simulink library "halin"  (R2021b)
settings: Solver=VariableStepAuto  StartTime=0.0  StopTime=10.0  RelTol=1e-3
undefined symbols (not defined in the file): KHAL_CAN1ABM1E2E_flg, KHAL_CAN1EPB1E2E_flg, KHAL_CAN1EPS1E2E_flg, KHAL_CAN1ESC1E2E_flg, KHAL_CAN1ESC5E2E_flg, KHAL_CAN3BMS1E2E_flg, KHAL_CAN3BMS6E2E_flg, KHAL_CAN3CCU1E2E_flg, KHAL_CAN3CCU2E2E_flg, KHAL_CAN3MCUNF1E2E_flg, KHAL_CAN3MCUNR1E2E_flg, KHAL_CAN3Shifter1E2E_flg, KHAL_CAN3Shifter2E2E_flg, KHAL_CAN6FCM2E2E_flg, KHAL_CAN6FCM4E2E_flg, TRUE
libraries: simulink x645, FVT_lib x207, hcu_lib x59
(part 13 of 23)

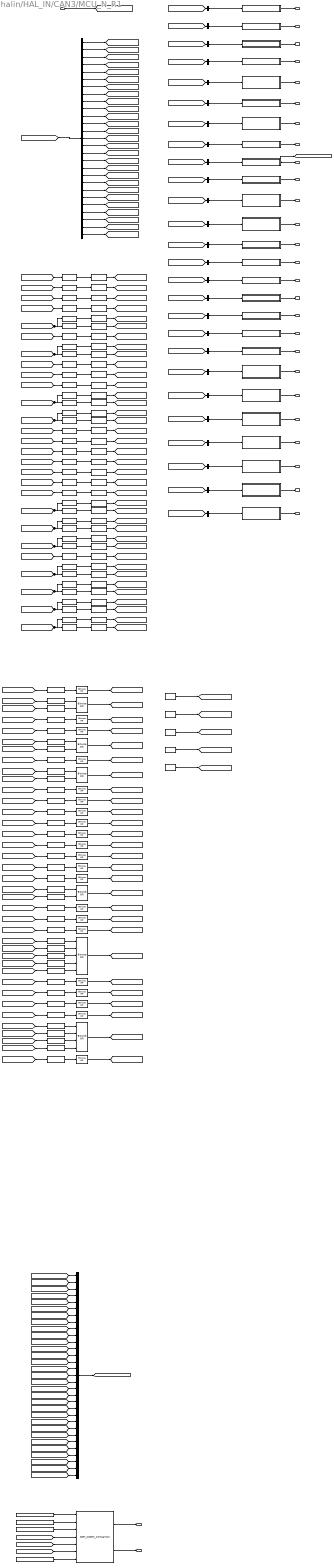
== system halin/HAL_IN/CAN3/MCU_N_R1 ==
  DT_CAN3_SG_MCU_N_R1 : Inport
  0x02 : Constant  Value=0x02
  0x78 : Constant  Value=0x78
  BitwiseAND{,1..37} (38 alike) : simulink/Logic and Bit Operations/Bitwise Operator  logicop=AND  UseBitMask=on  BitMask=0xFF  BitMaskRealWorld=Stored Integer
  BitwiseOR{,2..3,5,7..15,17..19,21..24,26} (21 alike) : simulink/Logic and Bit Operations/Bitwise Operator  logicop=OR  UseBitMask=off  BitMask=bin2dec('11011001')  BitMaskRealWorld=Stored Integer
  BitwiseOR{1,4,6,16} (4 alike) : simulink/Logic and Bit Operations/Bitwise Operator  logicop=OR  UseBitMask=off  NumInputPorts=2  BitMask=bin2dec('11011001')  BitMaskRealWorld=Stored Integer
  BitwiseOR20 : simulink/Logic and Bit Operations/Bitwise Operator  logicop=OR  UseBitMask=off  NumInputPorts=5  BitMask=bin2dec('11011001')  BitMaskRealWorld=Stored Integer
  BitwiseOR25 : simulink/Logic and Bit Operations/Bitwise Operator  logicop=OR  UseBitMask=off  NumInputPorts=4  BitMask=bin2dec('11011001')  BitMaskRealWorld=Stored Integer
  DDM_CS&RC_Comparison : FVT_lib/hal/DDM_CS&RC_Comparison  MsgCycleTime=10
  Data Type Conversion{,1..37} (38 alike) : DataTypeConversion  OutDataTypeStr=uint8
  KHAL_CAN3MCUNR1E2E_flg : Constant  Value=KHAL_CAN3MCUNR1E2E_flg
  LeftShift{,5,7,10..12,14} (7 alike) : ArithShift  BitShiftDirection=Left
  LeftShift1 : ArithShift  BitShiftNumber=1  BitShiftDirection=Left
  LeftShift13 : ArithShift  BitShiftNumber=7  BitShiftDirection=Left
  LeftShift15 : ArithShift  BitShiftNumber=1  BitShiftDirection=Left
  LeftShift2 : ArithShift  BitShiftNumber=2  BitShiftDirection=Left
  LeftShift3 : ArithShift  BitShiftNumber=5  BitShiftDirection=Left
  LeftShift4 : ArithShift  BitShiftNumber=6  BitShiftDirection=Left
  LeftShift6 : ArithShift  BitShiftNumber=4  BitShiftDirection=Left
  LeftShift8 : ArithShift  BitShiftNumber=3  BitShiftDirection=Left
  LeftShift9 : ArithShift  BitShiftNumber=4  BitShiftDirection=Left
  MCUWarnRNidec : Subsystem
  MessageRollingCounter : FVT_lib/hal/MessageRollingCounter  CounterMAX=14  task_time_ms=5  msg_time_ms=10
  Mux : Mux  Inputs=31
  RightShift{,2,4,6,10,14,16,18,20} (9 alike) : ArithShift  BitShiftNumber=8
  RightShift{1,3,5,7,11,15,17,19,21} (9 alike) : ArithShift
  RightShift12 : ArithShift  BitShiftNumber=4
  RightShift13 : ArithShift  BitShiftNumber=-4
  RightShift8 : ArithShift  BitShiftNumber=1
  RightShift9 : ArithShift  BitShiftNumber=-7
  RrActvDmpDisabStaNidec : Subsystem
  RrEDUDrtStaNidec : Subsystem
  RrEDUOpratingStaNidec : Subsystem
  RrEDURealTMTqNidec : Subsystem
  RrEDURotateDirctionNidec : Subsystem
  RrEDUTqReqFbkNidec : Subsystem
  RrMCU1ChksumNidec : Subsystem
  RrMCU1RolCntNidec : Subsystem
  RrMCUBATNidec : Subsystem
  RrMCUDCBusCurrNidec : Subsystem
  RrMCUDCBusVoltNidec : Subsystem
  RrMCUDischrgStaNidec : Subsystem
  RrMCUEnaStaNidec : Subsystem
  RrMCUErrNidec : Subsystem
  RrMCUIGNstaNidec : Subsystem
  RrMCUReady4PreNidec : Subsystem
  RrMCUReadyNidec : Subsystem
  RrMCUSysStaNidec : Subsystem
  RrMCUTempNidec : Subsystem
  RrMotorAvailTqNidec : Subsystem
  RrRegenAvailTqNidec : Subsystem
  RrTMSpdNidec : Subsystem
  RrTMTempNidec : Subsystem
  RrTMidNidec : Subsystem
  RrTMiqNidec : Subsystem
  bus_selector : BusSelector  OutputSignals=CAN3_MCUWarn_R_Nidec,CAN3_Rr_ActvDmpDisabSta_Nidec,CAN3_Rr_EDUDrtSta_Nidec,CAN3_Rr_EDUOpratingSta_Nidec,CAN3_Rr_EDURealTMTq_Nidec,CAN3_Rr_EDURotateDirction_Nidec,CAN3_Rr_EDUTqReqFbk_Nidec,CAN3_Rr_MCU1Chksum_Nidec,CAN3_Rr_MCU1RolCnt_Nidec,CAN3_Rr_MCUBAT_Nidec,CAN3_Rr_MCUDCBusCurr_Nidec,CAN3_Rr_MCUDCBusVolt_Nidec,CAN3_Rr_MCUDischrgSta_Nidec,CAN3_Rr_MCUEnaSta_Nidec,CAN3_Rr_MCUErr_Nidec,CAN3_Rr_MCUIGN_sta_Nidec,CAN3_Rr_MCUReady4Pre_Nidec,CAN3_Rr_MCUReady_Nidec,CAN3_Rr_MCUSysSta_Nidec,CAN3_Rr_MCUTemp_Nidec,CAN3_Rr_MotorAvailTq_Nidec,CAN3_Rr_RegenAvailTq_Nidec,CAN3_Rr_Reserved_bits_Nidec,CAN3_Rr_TMSpd_Nidec,CAN3_Rr_TMTemp_Nidec,CAN3_Rr_TMid_Nidec,CAN3_Rr_TMiq_Nidec
  bus_selector1 : BusSelector  OutputSignals=CAN3_MCUWarn_R_Nidec
  bus_selector10 : BusSelector  OutputSignals=CAN3_Rr_MCUBAT_Nidec
  bus_selector11 : BusSelector  OutputSignals=CAN3_Rr_MCUDCBusCurr_Nidec
  bus_selector12 : BusSelector  OutputSignals=CAN3_Rr_MCUDCBusVolt_Nidec
  bus_selector13 : BusSelector  OutputSignals=CAN3_Rr_MCUDischrgSta_Nidec
  bus_selector14 : BusSelector  OutputSignals=CAN3_Rr_MCUEnaSta_Nidec
  bus_selector15 : BusSelector  OutputSignals=CAN3_Rr_MCUErr_Nidec
  bus_selector16 : BusSelector  OutputSignals=CAN3_Rr_MCUIGN_sta_Nidec
  bus_selector17 : BusSelector  OutputSignals=CAN3_Rr_MCUReady4Pre_Nidec
  bus_selector18 : BusSelector  OutputSignals=CAN3_Rr_MCUReady_Nidec
  bus_selector19 : BusSelector  OutputSignals=CAN3_Rr_MCUSysSta_Nidec
  bus_selector2 : BusSelector  OutputSignals=CAN3_Rr_ActvDmpDisabSta_Nidec
  bus_selector20 : BusSelector  OutputSignals=CAN3_Rr_MCUTemp_Nidec
  bus_selector21 : BusSelector  OutputSignals=CAN3_Rr_MotorAvailTq_Nidec
  bus_selector22 : BusSelector  OutputSignals=CAN3_Rr_RegenAvailTq_Nidec
  bus_selector23 : BusSelector  OutputSignals=CAN3_Rr_TMSpd_Nidec
  bus_selector24 : BusSelector  OutputSignals=CAN3_Rr_TMTemp_Nidec
  bus_selector25 : BusSelector  OutputSignals=CAN3_Rr_TMid_Nidec
  bus_selector26 : BusSelector  OutputSignals=CAN3_Rr_TMiq_Nidec
  bus_selector3 : BusSelector  OutputSignals=CAN3_Rr_EDUDrtSta_Nidec
  bus_selector4 : BusSelector  OutputSignals=CAN3_Rr_EDUOpratingSta_Nidec
  bus_selector5 : BusSelector  OutputSignals=CAN3_Rr_EDURealTMTq_Nidec
  bus_selector6 : BusSelector  OutputSignals=CAN3_Rr_EDURotateDirction_Nidec
  bus_selector7 : BusSelector  OutputSignals=CAN3_Rr_EDUTqReqFbk_Nidec
  bus_selector8 : BusSelector  OutputSignals=CAN3_Rr_MCU1Chksum_Nidec
  bus_selector9 : BusSelector  OutputSignals=CAN3_Rr_MCU1RolCnt_Nidec
  constant{,1..4} (5 alike) : Constant  Value=0x0  OutDataTypeStr=uint8
  VHAL_MCUNR1CSErr_flg : Outport
  VHAL_MCUNR1RCErr_flg : Outport  Port=2
  VHAL_MCUWarnRNidec_enum : Outport  Port=3
  VHAL_RrActvDmpDisabStaNidec_flg : Outport  Port=4
  VHAL_RrEDUDrtStaNidec_flg : Outport  Port=5
  VHAL_RrEDUOpratingStaNidec_flg : Outport  Port=6
  VHAL_RrEDURealTMTqNidec_Nm : Outport  Port=7
  VHAL_RrEDURotateDirctionNidec_enum : Outport  Port=8
  VHAL_RrEDUTqReqFbkNidec_Nm : Outport  Port=9
  VHAL_RrMCU1ChksumNidec_enum : Outport  Port=10
  VHAL_RrMCU1RolCntNidec_enum : Outport  Port=11
  VHAL_RrMCUBATNidec_V : Outport  Port=12
  VHAL_RrMCUDCBusCurrNidec_A : Outport  Port=13
  VHAL_RrMCUDCBusVoltNidec_V : Outport  Port=14
  VHAL_RrMCUDischrgStaNidec_flg : Outport  Port=15
  VHAL_RrMCUEnaStaNidec_flg : Outport  Port=16
  VHAL_RrMCUErrNidec_enum : Outport  Port=17
  VHAL_RrMCUIGNstaNidec_flg : Outport  Port=18
  VHAL_RrMCUReady4PreNidec_flg : Outport  Port=19
  VHAL_RrMCUReadyNidec_flg : Outport  Port=20
  VHAL_RrMCUSysStaNidec_enum : Outport  Port=21
  VHAL_RrMCUTempNidec_C : Outport  Port=22
  VHAL_RrMotorAvailTqNidec_Nm : Outport  Port=23
  VHAL_RrRegenAvailTqNidec_Nm : Outport  Port=24
  VHAL_RrTMSpdNidec_rpm : Outport  Port=25
  VHAL_RrTMTempNidec_C : Outport  Port=26
  VHAL_RrTMidNidec_A : Outport  Port=27
  VHAL_RrTMiqNidec_A : Outport  Port=28
  wires:
  DT_CAN3_SG_MCU_N_R1/1 -> [DT_CAN3_SG_MCU_N_R1]
  [DT_CAN3_SG_MCU_N_R1] -> bus_selector/1
  bus_selector/1 -> [CAN3_MCUWarn_R_Nidec]  "<CAN3_MCUWarn_R_Nidec>"
  [CAN3_MCUWarn_R_Nidec] -> LeftShift/1
  LeftShift/1 -> BitwiseAND/1
  BitwiseAND/1 -> [Byte_1_CAN3_MCUWarn_R_Nidec]
  bus_selector/2 -> [CAN3_Rr_ActvDmpDisabSta_Nidec]  "<CAN3_Rr_ActvDmpDisabSta_Nidec>"
  [CAN3_Rr_ActvDmpDisabSta_Nidec] -> LeftShift1/1
  LeftShift1/1 -> BitwiseAND1/1
  BitwiseAND1/1 -> [Byte_25_CAN3_Rr_ActvDmpDisabSta_Nidec]
  bus_selector/3 -> [CAN3_Rr_EDUDrtSta_Nidec]  "<CAN3_Rr_EDUDrtSta_Nidec>"
  [CAN3_Rr_EDUDrtSta_Nidec] -> LeftShift2/1
  LeftShift2/1 -> BitwiseAND2/1
  BitwiseAND2/1 -> [Byte_25_CAN3_Rr_EDUDrtSta_Nidec]
  bus_selector/4 -> [CAN3_Rr_EDUOpratingSta_Nidec]  "<CAN3_Rr_EDUOpratingSta_Nidec>"
  [CAN3_Rr_EDUOpratingSta_Nidec] -> LeftShift3/1
  LeftShift3/1 -> BitwiseAND3/1
  BitwiseAND3/1 -> [Byte_30_CAN3_Rr_EDUOpratingSta_Nidec]
  bus_selector/5 -> [CAN3_Rr_EDURealTMTq_Nidec]  "<CAN3_Rr_EDURealTMTq_Nidec>"
  [CAN3_Rr_EDURealTMTq_Nidec] -> RightShift/1, RightShift1/1
  RightShift/1 -> BitwiseAND4/1
  BitwiseAND4/1 -> [Byte_28_CAN3_Rr_EDURealTMTq_Nidec]
  RightShift1/1 -> BitwiseAND5/1
  BitwiseAND5/1 -> [Byte_29_CAN3_Rr_EDURealTMTq_Nidec]
  bus_selector/6 -> [CAN3_Rr_EDURotateDirction_Nidec]  "<CAN3_Rr_EDURotateDirction_Nidec>"
  [CAN3_Rr_EDURotateDirction_Nidec] -> LeftShift4/1
  LeftShift4/1 -> BitwiseAND6/1
  BitwiseAND6/1 -> [Byte_30_CAN3_Rr_EDURotateDirction_Nidec]
  bus_selector/7 -> [CAN3_Rr_EDUTqReqFbk_Nidec]  "<CAN3_Rr_EDUTqReqFbk_Nidec>"
  [CAN3_Rr_EDUTqReqFbk_Nidec] -> RightShift2/1, RightShift3/1
  RightShift2/1 -> BitwiseAND7/1
  BitwiseAND7/1 -> [Byte_30_CAN3_Rr_EDUTqReqFbk_Nidec]
  RightShift3/1 -> BitwiseAND8/1
  BitwiseAND8/1 -> [Byte_31_CAN3_Rr_EDUTqReqFbk_Nidec]
  bus_selector/8 -> [CAN3_Rr_MCU1Chksum_Nidec]  "<CAN3_Rr_MCU1Chksum_Nidec>"
  [CAN3_Rr_MCU1Chksum_Nidec] -> LeftShift5/1
  LeftShift5/1 -> BitwiseAND9/1
  BitwiseAND9/1 -> [Byte_0_CAN3_Rr_MCU1Chksum_Nidec]
  bus_selector/9 -> [CAN3_Rr_MCU1RolCnt_Nidec]  "<CAN3_Rr_MCU1RolCnt_Nidec>"
  [CAN3_Rr_MCU1RolCnt_Nidec] -> LeftShift6/1
  LeftShift6/1 -> BitwiseAND10/1
  BitwiseAND10/1 -> [Byte_1_CAN3_Rr_MCU1RolCnt_Nidec]
  bus_selector/10 -> [CAN3_Rr_MCUBAT_Nidec]  "<CAN3_Rr_MCUBAT_Nidec>"
  [CAN3_Rr_MCUBAT_Nidec] -> LeftShift7/1
  LeftShift7/1 -> BitwiseAND11/1
  BitwiseAND11/1 -> [Byte_8_CAN3_Rr_MCUBAT_Nidec]
  bus_selector/11 -> [CAN3_Rr_MCUDCBusCurr_Nidec]  "<CAN3_Rr_MCUDCBusCurr_Nidec>"
  [CAN3_Rr_MCUDCBusCurr_Nidec] -> RightShift4/1, RightShift5/1
  RightShift4/1 -> BitwiseAND12/1
  BitwiseAND12/1 -> [Byte_21_CAN3_Rr_MCUDCBusCurr_Nidec]
  RightShift5/1 -> BitwiseAND13/1
  BitwiseAND13/1 -> [Byte_22_CAN3_Rr_MCUDCBusCurr_Nidec]
  bus_selector/12 -> [CAN3_Rr_MCUDCBusVolt_Nidec]  "<CAN3_Rr_MCUDCBusVolt_Nidec>"
  [CAN3_Rr_MCUDCBusVolt_Nidec] -> RightShift6/1, RightShift7/1
  RightShift6/1 -> BitwiseAND14/1
  BitwiseAND14/1 -> [Byte_23_CAN3_Rr_MCUDCBusVolt_Nidec]
  RightShift7/1 -> BitwiseAND15/1
  BitwiseAND15/1 -> [Byte_24_CAN3_Rr_MCUDCBusVolt_Nidec]
  bus_selector/13 -> [CAN3_Rr_MCUDischrgSta_Nidec]  "<CAN3_Rr_MCUDischrgSta_Nidec>"
  [CAN3_Rr_MCUDischrgSta_Nidec] -> LeftShift8/1
  LeftShift8/1 -> BitwiseAND16/1
  BitwiseAND16/1 -> [Byte_25_CAN3_Rr_MCUDischrgSta_Nidec]
  bus_selector/14 -> [CAN3_Rr_MCUEnaSta_Nidec]  "<CAN3_Rr_MCUEnaSta_Nidec>"
  [CAN3_Rr_MCUEnaSta_Nidec] -> LeftShift9/1
  LeftShift9/1 -> BitwiseAND17/1
  BitwiseAND17/1 -> [Byte_30_CAN3_Rr_MCUEnaSta_Nidec]
  bus_selector/15 -> [CAN3_Rr_MCUErr_Nidec]  "<CAN3_Rr_MCUErr_Nidec>"
  [CAN3_Rr_MCUErr_Nidec] -> LeftShift10/1
  LeftShift10/1 -> BitwiseAND18/1
  BitwiseAND18/1 -> [Byte_17_CAN3_Rr_MCUErr_Nidec]
  bus_selector/16 -> [CAN3_Rr_MCUIGN_sta_Nidec]  "<CAN3_Rr_MCUIGN_sta_Nidec>"
  [CAN3_Rr_MCUIGN_sta_Nidec] -> LeftShift11/1
  LeftShift11/1 -> BitwiseAND19/1
  BitwiseAND19/1 -> [Byte_9_CAN3_Rr_MCUIGN_sta_Nidec]
  bus_selector/17 -> [CAN3_Rr_MCUReady4Pre_Nidec]  "<CAN3_Rr_MCUReady4Pre_Nidec>"
  [CAN3_Rr_MCUReady4Pre_Nidec] -> LeftShift12/1
  LeftShift12/1 -> BitwiseAND20/1
  BitwiseAND20/1 -> [Byte_25_CAN3_Rr_MCUReady4Pre_Nidec]
  bus_selector/18 -> [CAN3_Rr_MCUReady_Nidec]  "<CAN3_Rr_MCUReady_Nidec>"
  [CAN3_Rr_MCUReady_Nidec] -> LeftShift13/1
  LeftShift13/1 -> BitwiseAND21/1
  BitwiseAND21/1 -> [Byte_25_CAN3_Rr_MCUReady_Nidec]
  bus_selector/19 -> [CAN3_Rr_MCUSysSta_Nidec]  "<CAN3_Rr_MCUSysSta_Nidec>"
  [CAN3_Rr_MCUSysSta_Nidec] -> LeftShift14/1
  LeftShift14/1 -> BitwiseAND22/1
  BitwiseAND22/1 -> [Byte_7_CAN3_Rr_MCUSysSta_Nidec]
  bus_selector/20 -> [CAN3_Rr_MCUTemp_Nidec]  "<CAN3_Rr_MCUTemp_Nidec>"
  [CAN3_Rr_MCUTemp_Nidec] -> RightShift8/1, RightShift9/1
  RightShift8/1 -> BitwiseAND23/1
  BitwiseAND23/1 -> [Byte_20_CAN3_Rr_MCUTemp_Nidec]
  RightShift9/1 -> BitwiseAND24/1
  BitwiseAND24/1 -> [Byte_21_CAN3_Rr_MCUTemp_Nidec]
  bus_selector/21 -> [CAN3_Rr_MotorAvailTq_Nidec]  "<CAN3_Rr_MotorAvailTq_Nidec>"
  [CAN3_Rr_MotorAvailTq_Nidec] -> RightShift10/1, RightShift11/1
  RightShift10/1 -> BitwiseAND25/1
  BitwiseAND25/1 -> [Byte_11_CAN3_Rr_MotorAvailTq_Nidec]
  RightShift11/1 -> BitwiseAND26/1
  BitwiseAND26/1 -> [Byte_12_CAN3_Rr_MotorAvailTq_Nidec]
  bus_selector/22 -> [CAN3_Rr_RegenAvailTq_Nidec]  "<CAN3_Rr_RegenAvailTq_Nidec>"
  [CAN3_Rr_RegenAvailTq_Nidec] -> RightShift12/1, RightShift13/1
  RightShift12/1 -> BitwiseAND27/1
  BitwiseAND27/1 -> [Byte_10_CAN3_Rr_RegenAvailTq_Nidec]
  RightShift13/1 -> BitwiseAND28/1
  BitwiseAND28/1 -> [Byte_11_CAN3_Rr_RegenAvailTq_Nidec]
  bus_selector/23 -> [CAN3_Rr_Reserved_bits_Nidec]  "<CAN3_Rr_Reserved_bits_Nidec>"
  [CAN3_Rr_Reserved_bits_Nidec] -> LeftShift15/1
  LeftShift15/1 -> BitwiseAND29/1
  BitwiseAND29/1 -> [Byte_9_CAN3_Rr_Reserved_bits_Nidec]
  bus_selector/24 -> [CAN3_Rr_TMSpd_Nidec]  "<CAN3_Rr_TMSpd_Nidec>"
  [CAN3_Rr_TMSpd_Nidec] -> RightShift14/1, RightShift15/1
  RightShift14/1 -> BitwiseAND30/1
  BitwiseAND30/1 -> [Byte_26_CAN3_Rr_TMSpd_Nidec]
  RightShift15/1 -> BitwiseAND31/1
  BitwiseAND31/1 -> [Byte_27_CAN3_Rr_TMSpd_Nidec]
  bus_selector/25 -> [CAN3_Rr_TMTemp_Nidec]  "<CAN3_Rr_TMTemp_Nidec>"
  [CAN3_Rr_TMTemp_Nidec] -> RightShift16/1, RightShift17/1
  RightShift16/1 -> BitwiseAND32/1
  BitwiseAND32/1 -> [Byte_18_CAN3_Rr_TMTemp_Nidec]
  RightShift17/1 -> BitwiseAND33/1
  BitwiseAND33/1 -> [Byte_19_CAN3_Rr_TMTemp_Nidec]
  bus_selector/26 -> [CAN3_Rr_TMid_Nidec]  "<CAN3_Rr_TMid_Nidec>"
  [CAN3_Rr_TMid_Nidec] -> RightShift18/1, RightShift19/1
  RightShift18/1 -> BitwiseAND34/1
  BitwiseAND34/1 -> [Byte_15_CAN3_Rr_TMid_Nidec]
  RightShift19/1 -> BitwiseAND35/1
  BitwiseAND35/1 -> [Byte_16_CAN3_Rr_TMid_Nidec]
  bus_selector/27 -> [CAN3_Rr_TMiq_Nidec]  "<CAN3_Rr_TMiq_Nidec>"
  [CAN3_Rr_TMiq_Nidec] -> RightShift20/1, RightShift21/1
  RightShift20/1 -> BitwiseAND36/1
  BitwiseAND36/1 -> [Byte_13_CAN3_Rr_TMiq_Nidec]
  RightShift21/1 -> BitwiseAND37/1
  BitwiseAND37/1 -> [Byte_14_CAN3_Rr_TMiq_Nidec]
  Data Type Conversion/1 -> BitwiseOR/1
  [Byte_0_CAN3_Rr_MCU1Chksum_Nidec] -> Data Type Conversion/1
  BitwiseOR/1 -> [Byte_0]
  Data Type Conversion1/1 -> BitwiseOR1/1
  [Byte_1_CAN3_MCUWarn_R_Nidec] -> Data Type Conversion1/1
  Data Type Conversion2/1 -> BitwiseOR1/2
  [Byte_1_CAN3_Rr_MCU1RolCnt_Nidec] -> Data Type Conversion2/1
  BitwiseOR1/1 -> [Byte_1]
  constant/1 -> [Byte_2]
  constant1/1 -> [Byte_3]
  constant2/1 -> [Byte_4]
  constant3/1 -> [Byte_5]
  constant4/1 -> [Byte_6]
  Data Type Conversion3/1 -> BitwiseOR2/1
  [Byte_7_CAN3_Rr_MCUSysSta_Nidec] -> Data Type Conversion3/1
  BitwiseOR2/1 -> [Byte_7]
  Data Type Conversion4/1 -> BitwiseOR3/1
  [Byte_8_CAN3_Rr_MCUBAT_Nidec] -> Data Type Conversion4/1
  BitwiseOR3/1 -> [Byte_8]
  Data Type Conversion5/1 -> BitwiseOR4/1
  [Byte_9_CAN3_Rr_MCUIGN_sta_Nidec] -> Data Type Conversion5/1
  Data Type Conversion6/1 -> BitwiseOR4/2
  [Byte_9_CAN3_Rr_Reserved_bits_Nidec] -> Data Type Conversion6/1
  BitwiseOR4/1 -> [Byte_9]
  Data Type Conversion7/1 -> BitwiseOR5/1
  [Byte_10_CAN3_Rr_RegenAvailTq_Nidec] -> Data Type Conversion7/1
  BitwiseOR5/1 -> [Byte_10]
  Data Type Conversion8/1 -> BitwiseOR6/1
  [Byte_11_CAN3_Rr_MotorAvailTq_Nidec] -> Data Type Conversion8/1
  Data Type Conversion9/1 -> BitwiseOR6/2
  [Byte_11_CAN3_Rr_RegenAvailTq_Nidec] -> Data Type Conversion9/1
  BitwiseOR6/1 -> [Byte_11]
  Data Type Conversion10/1 -> BitwiseOR7/1
  [Byte_12_CAN3_Rr_MotorAvailTq_Nidec] -> Data Type Conversion10/1
  BitwiseOR7/1 -> [Byte_12]
  Data Type Conversion11/1 -> BitwiseOR8/1
  [Byte_13_CAN3_Rr_TMiq_Nidec] -> Data Type Conversion11/1
  BitwiseOR8/1 -> [Byte_13]
  Data Type Conversion12/1 -> BitwiseOR9/1
  [Byte_14_CAN3_Rr_TMiq_Nidec] -> Data Type Conversion12/1
  BitwiseOR9/1 -> [Byte_14]
  Data Type Conversion13/1 -> BitwiseOR10/1
  [Byte_15_CAN3_Rr_TMid_Nidec] -> Data Type Conversion13/1
  BitwiseOR10/1 -> [Byte_15]
  Data Type Conversion14/1 -> BitwiseOR11/1
  [Byte_16_CAN3_Rr_TMid_Nidec] -> Data Type Conversion14/1
  BitwiseOR11/1 -> [Byte_16]
  Data Type Conversion15/1 -> BitwiseOR12/1
  [Byte_17_CAN3_Rr_MCUErr_Nidec] -> Data Type Conversion15/1
  BitwiseOR12/1 -> [Byte_17]
  Data Type Conversion16/1 -> BitwiseOR13/1
  [Byte_18_CAN3_Rr_TMTemp_Nidec] -> Data Type Conversion16/1
  BitwiseOR13/1 -> [Byte_18]
  Data Type Conversion17/1 -> BitwiseOR14/1
  [Byte_19_CAN3_Rr_TMTemp_Nidec] -> Data Type Conversion17/1
  BitwiseOR14/1 -> [Byte_19]
  Data Type Conversion18/1 -> BitwiseOR15/1
  [Byte_20_CAN3_Rr_MCUTemp_Nidec] -> Data Type Conversion18/1
  BitwiseOR15/1 -> [Byte_20]
  Data Type Conversion19/1 -> BitwiseOR16/1
  [Byte_21_CAN3_Rr_MCUDCBusCurr_Nidec] -> Data Type Conversion19/1
  Data Type Conversion20/1 -> BitwiseOR16/2
  [Byte_21_CAN3_Rr_MCUTemp_Nidec] -> Data Type Conversion20/1
  BitwiseOR16/1 -> [Byte_21]
  Data Type Conversion21/1 -> BitwiseOR17/1
  [Byte_22_CAN3_Rr_MCUDCBusCurr_Nidec] -> Data Type Conversion21/1
  BitwiseOR17/1 -> [Byte_22]
  Data Type Conversion22/1 -> BitwiseOR18/1
  [Byte_23_CAN3_Rr_MCUDCBusVolt_Nidec] -> Data Type Conversion22/1
  BitwiseOR18/1 -> [Byte_23]
  Data Type Conversion23/1 -> BitwiseOR19/1
  [Byte_24_CAN3_Rr_MCUDCBusVolt_Nidec] -> Data Type Conversion23/1
  BitwiseOR19/1 -> [Byte_24]
  Data Type Conversion24/1 -> BitwiseOR20/1
  [Byte_25_CAN3_Rr_ActvDmpDisabSta_Nidec] -> Data Type Conversion24/1
  Data Type Conversion25/1 -> BitwiseOR20/2
  [Byte_25_CAN3_Rr_EDUDrtSta_Nidec] -> Data Type Conversion25/1
  Data Type Conversion26/1 -> BitwiseOR20/3
  [Byte_25_CAN3_Rr_MCUDischrgSta_Nidec] -> Data Type Conversion26/1
  Data Type Conversion27/1 -> BitwiseOR20/4
  [Byte_25_CAN3_Rr_MCUReady4Pre_Nidec] -> Data Type Conversion27/1
  Data Type Conversion28/1 -> BitwiseOR20/5
  [Byte_25_CAN3_Rr_MCUReady_Nidec] -> Data Type Conversion28/1
  BitwiseOR20/1 -> [Byte_25]
  Data Type Conversion29/1 -> BitwiseOR21/1
  [Byte_26_CAN3_Rr_TMSpd_Nidec] -> Data Type Conversion29/1
  BitwiseOR21/1 -> [Byte_26]
  Data Type Conversion30/1 -> BitwiseOR22/1
  [Byte_27_CAN3_Rr_TMSpd_Nidec] -> Data Type Conversion30/1
  BitwiseOR22/1 -> [Byte_27]
  Data Type Conversion31/1 -> BitwiseOR23/1
  [Byte_28_CAN3_Rr_EDURealTMTq_Nidec] -> Data Type Conversion31/1
  BitwiseOR23/1 -> [Byte_28]
  Data Type Conversion32/1 -> BitwiseOR24/1
  [Byte_29_CAN3_Rr_EDURealTMTq_Nidec] -> Data Type Conversion32/1
  BitwiseOR24/1 -> [Byte_29]
  Data Type Conversion33/1 -> BitwiseOR25/1
  [Byte_30_CAN3_Rr_EDUOpratingSta_Nidec] -> Data Type Conversion33/1
  Data Type Conversion34/1 -> BitwiseOR25/2
  [Byte_30_CAN3_Rr_EDURotateDirction_Nidec] -> Data Type Conversion34/1
  Data Type Conversion35/1 -> BitwiseOR25/3
  [Byte_30_CAN3_Rr_EDUTqReqFbk_Nidec] -> Data Type Conversion35/1
  Data Type Conversion36/1 -> BitwiseOR25/4
  [Byte_30_CAN3_Rr_MCUEnaSta_Nidec] -> Data Type Conversion36/1
  BitwiseOR25/1 -> [Byte_30]
  Data Type Conversion37/1 -> BitwiseOR26/1
  [Byte_31_CAN3_Rr_EDUTqReqFbk_Nidec] -> Data Type Conversion37/1
  BitwiseOR26/1 -> [Byte_31]
  [Byte_1] -> Mux/1
  [Byte_2] -> Mux/2
  [Byte_3] -> Mux/3
  [Byte_4] -> Mux/4
  [Byte_5] -> Mux/5
  [Byte_6] -> Mux/6
  [Byte_7] -> Mux/7
  [Byte_8] -> Mux/8
  [Byte_9] -> Mux/9
  [Byte_10] -> Mux/10
  [Byte_11] -> Mux/11
  [Byte_12] -> Mux/12
  [Byte_13] -> Mux/13
  [Byte_14] -> Mux/14
  [Byte_15] -> Mux/15
  [Byte_16] -> Mux/16
  [Byte_17] -> Mux/17
  [Byte_18] -> Mux/18
  [Byte_19] -> Mux/19
  [Byte_20] -> Mux/20
  [Byte_21] -> Mux/21
  [Byte_22] -> Mux/22
  [Byte_23] -> Mux/23
  [Byte_24] -> Mux/24
  [Byte_25] -> Mux/25
  [Byte_26] -> Mux/26
  [Byte_27] -> Mux/27
  [Byte_28] -> Mux/28
  [Byte_29] -> Mux/29
  [Byte_30] -> Mux/30
  [Byte_31] -> Mux/31
  Mux/1 -> [VHAL_CAN3MCUNR1noCS_raw]
  KHAL_CAN3MCUNR1E2E_flg/1 -> DDM_CS&RC_Comparison/1
  0x78/1 -> DDM_CS&RC_Comparison/2
  0x02/1 -> DDM_CS&RC_Comparison/3
  [VHAL_CAN3MCUNR1noCS_raw] -> DDM_CS&RC_Comparison/4
  [Byte_0] -> DDM_CS&RC_Comparison/5
  [RC_ECU] -> DDM_CS&RC_Comparison/6
  MessageRollingCounter/1 -> DDM_CS&RC_Comparison/7
  DDM_CS&RC_Comparison/1 -> VHAL_MCUNR1CSErr_flg/1
  DDM_CS&RC_Comparison/2 -> VHAL_MCUNR1RCErr_flg/1
  [DT_CAN3_SG_MCU_N_R1] -> bus_selector1/1
  bus_selector1/1 -> MCUWarnRNidec/1(MCUWarn_R_Nidec)  "<CAN3_MCUWarn_R_Nidec>"
  MCUWarnRNidec/1(VHAL_MCUWarnRNidec_enum) -> VHAL_MCUWarnRNidec_enum/1
  [DT_CAN3_SG_MCU_N_R1] -> bus_selector2/1
  bus_selector2/1 -> RrActvDmpDisabStaNidec/1(Rr_ActvDmpDisabSta_Nidec)  "<CAN3_Rr_ActvDmpDisabSta_Nidec>"
  RrActvDmpDisabStaNidec/1(VHAL_RrActvDmpDisabStaNidec_flg) -> VHAL_RrActvDmpDisabStaNidec_flg/1
  [DT_CAN3_SG_MCU_N_R1] -> bus_selector3/1
  bus_selector3/1 -> RrEDUDrtStaNidec/1(Rr_EDUDrtSta_Nidec)  "<CAN3_Rr_EDUDrtSta_Nidec>"
  RrEDUDrtStaNidec/1(VHAL_RrEDUDrtStaNidec_flg) -> VHAL_RrEDUDrtStaNidec_flg/1
  [DT_CAN3_SG_MCU_N_R1] -> bus_selector4/1
  bus_selector4/1 -> RrEDUOpratingStaNidec/1(Rr_EDUOpratingSta_Nidec)  "<CAN3_Rr_EDUOpratingSta_Nidec>"
  RrEDUOpratingStaNidec/1(VHAL_RrEDUOpratingStaNidec_flg) -> VHAL_RrEDUOpratingStaNidec_flg/1
  [DT_CAN3_SG_MCU_N_R1] -> bus_selector5/1
  bus_selector5/1 -> RrEDURealTMTqNidec/1(Rr_EDURealTMTq_Nidec)  "<CAN3_Rr_EDURealTMTq_Nidec>"
  RrEDURealTMTqNidec/1(VHAL_RrEDURealTMTqNidec_Nm) -> VHAL_RrEDURealTMTqNidec_Nm/1
  [DT_CAN3_SG_MCU_N_R1] -> bus_selector6/1
  bus_selector6/1 -> RrEDURotateDirctionNidec/1(Rr_EDURotateDirction_Nidec)  "<CAN3_Rr_EDURotateDirction_Nidec>"
  RrEDURotateDirctionNidec/1(VHAL_RrEDURotateDirctionNidec_enum) -> VHAL_RrEDURotateDirctionNidec_enum/1
  [DT_CAN3_SG_MCU_N_R1] -> bus_selector7/1
  bus_selector7/1 -> RrEDUTqReqFbkNidec/1(Rr_EDUTqReqFbk_Nidec)  "<CAN3_Rr_EDUTqReqFbk_Nidec>"
  RrEDUTqReqFbkNidec/1(VHAL_RrEDUTqReqFbkNidec_Nm) -> VHAL_RrEDUTqReqFbkNidec_Nm/1
  [DT_CAN3_SG_MCU_N_R1] -> bus_selector8/1
  bus_selector8/1 -> RrMCU1ChksumNidec/1(Rr_MCU1Chksum_Nidec)  "<CAN3_Rr_MCU1Chksum_Nidec>"
  RrMCU1ChksumNidec/1(VHAL_RrMCU1ChksumNidec_enum) -> VHAL_RrMCU1ChksumNidec_enum/1
  [DT_CAN3_SG_MCU_N_R1] -> bus_selector9/1
  bus_selector9/1 -> RrMCU1RolCntNidec/1(Rr_MCU1RolCnt_Nidec)  "<CAN3_Rr_MCU1RolCnt_Nidec>"
  RrMCU1RolCntNidec/1(VHAL_RrMCU1RolCntNidec_enum) -> VHAL_RrMCU1RolCntNidec_enum/1, [RC_ECU]
  [DT_CAN3_SG_MCU_N_R1] -> bus_selector10/1
  bus_selector10/1 -> RrMCUBATNidec/1(Rr_MCUBAT_Nidec)  "<CAN3_Rr_MCUBAT_Nidec>"
  RrMCUBATNidec/1(VHAL_RrMCUBATNidec_V) -> VHAL_RrMCUBATNidec_V/1
  [DT_CAN3_SG_MCU_N_R1] -> bus_selector11/1
  bus_selector11/1 -> RrMCUDCBusCurrNidec/1(Rr_MCUDCBusCurr_Nidec)  "<CAN3_Rr_MCUDCBusCurr_Nidec>"
  RrMCUDCBusCurrNidec/1(VHAL_RrMCUDCBusCurrNidec_A) -> VHAL_RrMCUDCBusCurrNidec_A/1
  [DT_CAN3_SG_MCU_N_R1] -> bus_selector12/1
  bus_selector12/1 -> RrMCUDCBusVoltNidec/1(Rr_MCUDCBusVolt_Nidec)  "<CAN3_Rr_MCUDCBusVolt_Nidec>"
  RrMCUDCBusVoltNidec/1(VHAL_RrMCUDCBusVoltNidec_V) -> VHAL_RrMCUDCBusVoltNidec_V/1
  [DT_CAN3_SG_MCU_N_R1] -> bus_selector13/1
  bus_selector13/1 -> RrMCUDischrgStaNidec/1(Rr_MCUDischrgSta_Nidec)  "<CAN3_Rr_MCUDischrgSta_Nidec>"
  RrMCUDischrgStaNidec/1(VHAL_RrMCUDischrgStaNidec_flg) -> VHAL_RrMCUDischrgStaNidec_flg/1
  [DT_CAN3_SG_MCU_N_R1] -> bus_selector14/1
  bus_selector14/1 -> RrMCUEnaStaNidec/1(Rr_MCUEnaSta_Nidec)  "<CAN3_Rr_MCUEnaSta_Nidec>"
  RrMCUEnaStaNidec/1(VHAL_RrMCUEnaStaNidec_flg) -> VHAL_RrMCUEnaStaNidec_flg/1
  [DT_CAN3_SG_MCU_N_R1] -> bus_selector15/1
  bus_selector15/1 -> RrMCUErrNidec/1(Rr_MCUErr_Nidec)  "<CAN3_Rr_MCUErr_Nidec>"
  RrMCUErrNidec/1(VHAL_RrMCUErrNidec_enum) -> VHAL_RrMCUErrNidec_enum/1
  [DT_CAN3_SG_MCU_N_R1] -> bus_selector16/1
  bus_selector16/1 -> RrMCUIGNstaNidec/1(Rr_MCUIGN_sta_Nidec)  "<CAN3_Rr_MCUIGN_sta_Nidec>"
  RrMCUIGNstaNidec/1(VHAL_RrMCUIGNstaNidec_flg) -> VHAL_RrMCUIGNstaNidec_flg/1
  [DT_CAN3_SG_MCU_N_R1] -> bus_selector17/1
  bus_selector17/1 -> RrMCUReady4PreNidec/1(Rr_MCUReady4Pre_Nidec)  "<CAN3_Rr_MCUReady4Pre_Nidec>"
  RrMCUReady4PreNidec/1(VHAL_RrMCUReady4PreNidec_flg) -> VHAL_RrMCUReady4PreNidec_flg/1
  [DT_CAN3_SG_MCU_N_R1] -> bus_selector18/1
  bus_selector18/1 -> RrMCUReadyNidec/1(Rr_MCUReady_Nidec)  "<CAN3_Rr_MCUReady_Nidec>"
  RrMCUReadyNidec/1(VHAL_RrMCUReadyNidec_flg) -> VHAL_RrMCUReadyNidec_flg/1
  [DT_CAN3_SG_MCU_N_R1] -> bus_selector19/1
  bus_selector19/1 -> RrMCUSysStaNidec/1(Rr_MCUSysSta_Nidec)  "<CAN3_Rr_MCUSysSta_Nidec>"
  RrMCUSysStaNidec/1(VHAL_RrMCUSysStaNidec_enum) -> VHAL_RrMCUSysStaNidec_enum/1
  [DT_CAN3_SG_MCU_N_R1] -> bus_selector20/1
  bus_selector20/1 -> RrMCUTempNidec/1(Rr_MCUTemp_Nidec)  "<CAN3_Rr_MCUTemp_Nidec>"
  RrMCUTempNidec/1(VHAL_RrMCUTempNidec_C) -> VHAL_RrMCUTempNidec_C/1
  [DT_CAN3_SG_MCU_N_R1] -> bus_selector21/1
  bus_selector21/1 -> RrMotorAvailTqNidec/1(Rr_MotorAvailTq_Nidec)  "<CAN3_Rr_MotorAvailTq_Nidec>"
  RrMotorAvailTqNidec/1(VHAL_RrMotorAvailTqNidec_Nm) -> VHAL_RrMotorAvailTqNidec_Nm/1
  [DT_CAN3_SG_MCU_N_R1] -> bus_selector22/1
  bus_selector22/1 -> RrRegenAvailTqNidec/1(Rr_RegenAvailTq_Nidec)  "<CAN3_Rr_RegenAvailTq_Nidec>"
  RrRegenAvailTqNidec/1(VHAL_RrRegenAvailTqNidec_Nm) -> VHAL_RrRegenAvailTqNidec_Nm/1
  [DT_CAN3_SG_MCU_N_R1] -> bus_selector23/1
  bus_selector23/1 -> RrTMSpdNidec/1(Rr_TMSpd_Nidec)  "<CAN3_Rr_TMSpd_Nidec>"
  RrTMSpdNidec/1(VHAL_RrTMSpdNidec_rpm) -> VHAL_RrTMSpdNidec_rpm/1
  [DT_CAN3_SG_MCU_N_R1] -> bus_selector24/1
  bus_selector24/1 -> RrTMTempNidec/1(Rr_TMTemp_Nidec)  "<CAN3_Rr_TMTemp_Nidec>"
  RrTMTempNidec/1(VHAL_RrTMTempNidec_C) -> VHAL_RrTMTempNidec_C/1
  [DT_CAN3_SG_MCU_N_R1] -> bus_selector25/1
  bus_selector25/1 -> RrTMidNidec/1(Rr_TMid_Nidec)  "<CAN3_Rr_TMid_Nidec>"
  RrTMidNidec/1(VHAL_RrTMidNidec_A) -> VHAL_RrTMidNidec_A/1
  [DT_CAN3_SG_MCU_N_R1] -> bus_selector26/1
  bus_selector26/1 -> RrTMiqNidec/1(Rr_TMiq_Nidec)  "<CAN3_Rr_TMiq_Nidec>"
  RrTMiqNidec/1(VHAL_RrTMiqNidec_A) -> VHAL_RrTMiqNidec_A/1

== system halin/HAL_IN/CAN3/MCU_N_R2 ==
  DT_CAN3_SG_MCU_N_R2 : Inport
  RrCoolanttempReqNidec : Subsystem
  RrEOPSpdSetNidec : Subsystem
  RrFailcode1Nidec : Subsystem
  RrFailcode2Nidec : Subsystem
  RrFailcodehistory1Nidec : Subsystem
  RrFailcodehistory2Nidec : Subsystem
  RrLLCTempNidec : Subsystem
  RrLLCflowReqNidec : Subsystem
  RrMCUTempWarnNidec : Subsystem
  RrTMTempWarnNidec : Subsystem
  bus_selector : BusSelector  OutputSignals=CAN3_Rr_CoolanttempReq_Nidec
  bus_selector1 : BusSelector  OutputSignals=CAN3_Rr_EOP_SpdSet_Nidec
  bus_selector2 : BusSelector  OutputSignals=CAN3_Rr_Failcode1_Nidec
  bus_selector3 : BusSelector  OutputSignals=CAN3_Rr_Failcode2_Nidec
  bus_selector4 : BusSelector  OutputSignals=CAN3_Rr_Failcodehistory1_Nidec
  bus_selector5 : BusSelector  OutputSignals=CAN3_Rr_Failcodehistory2_Nidec
  bus_selector6 : BusSelector  OutputSignals=CAN3_Rr_LLCTemp_Nidec
  bus_selector7 : BusSelector  OutputSignals=CAN3_Rr_LLCflowReq_Nidec
  bus_selector8 : BusSelector  OutputSignals=CAN3_Rr_MCUTempWarn_Nidec
  bus_selector9 : BusSelector  OutputSignals=CAN3_Rr_TMTempWarn_Nidec
  VHAL_RrCoolanttempReqNidec_cnt : Outport
  VHAL_RrEOPSpdSetNidec_rpm : Outport  Port=2
  VHAL_RrFailcode1Nidec_enum : Outport  Port=3
  VHAL_RrFailcode2Nidec_enum : Outport  Port=4
  VHAL_RrFailcodehistory1Nidec_enum : Outport  Port=5
  VHAL_RrFailcodehistory2Nidec_enum : Outport  Port=6
  VHAL_RrLLCTempNidec_C : Outport  Port=7
  VHAL_RrLLCflowReqNidec_Lpmin : Outport  Port=8
  VHAL_RrMCUTempWarnNidec_enum : Outport  Port=9
  VHAL_RrTMTempWarnNidec_enum : Outport  Port=10
  wires:
  DT_CAN3_SG_MCU_N_R2/1 -> [DT_CAN3_SG_MCU_N_R2]
  [DT_CAN3_SG_MCU_N_R2] -> bus_selector/1
  bus_selector/1 -> RrCoolanttempReqNidec/1(Rr_CoolanttempReq_Nidec)  "<CAN3_Rr_CoolanttempReq_Nidec>"
  RrCoolanttempReqNidec/1(VHAL_RrCoolanttempReqNidec_cnt) -> VHAL_RrCoolanttempReqNidec_cnt/1
  [DT_CAN3_SG_MCU_N_R2] -> bus_selector1/1
  bus_selector1/1 -> RrEOPSpdSetNidec/1(Rr_EOP_SpdSet_Nidec)  "<CAN3_Rr_EOP_SpdSet_Nidec>"
  RrEOPSpdSetNidec/1(VHAL_RrEOPSpdSetNidec_rpm) -> VHAL_RrEOPSpdSetNidec_rpm/1
  [DT_CAN3_SG_MCU_N_R2] -> bus_selector2/1
  bus_selector2/1 -> RrFailcode1Nidec/1(Rr_Failcode1_Nidec)  "<CAN3_Rr_Failcode1_Nidec>"
  RrFailcode1Nidec/1(VHAL_RrFailcode1Nidec_enum) -> VHAL_RrFailcode1Nidec_enum/1
  [DT_CAN3_SG_MCU_N_R2] -> bus_selector3/1
  bus_selector3/1 -> RrFailcode2Nidec/1(Rr_Failcode2_Nidec)  "<CAN3_Rr_Failcode2_Nidec>"
  RrFailcode2Nidec/1(VHAL_RrFailcode2Nidec_enum) -> VHAL_RrFailcode2Nidec_enum/1
  [DT_CAN3_SG_MCU_N_R2] -> bus_selector4/1
  bus_selector4/1 -> RrFailcodehistory1Nidec/1(Rr_Failcodehistory1_Nidec)  "<CAN3_Rr_Failcodehistory1_Nidec>"
  RrFailcodehistory1Nidec/1(VHAL_RrFailcodehistory1Nidec_enum) -> VHAL_RrFailcodehistory1Nidec_enum/1
  [DT_CAN3_SG_MCU_N_R2] -> bus_selector5/1
  bus_selector5/1 -> RrFailcodehistory2Nidec/1(Rr_Failcodehistory2_Nidec)  "<CAN3_Rr_Failcodehistory2_Nidec>"
  RrFailcodehistory2Nidec/1(VHAL_RrFailcodehistory2Nidec_enum) -> VHAL_RrFailcodehistory2Nidec_enum/1
  [DT_CAN3_SG_MCU_N_R2] -> bus_selector6/1
  bus_selector6/1 -> RrLLCTempNidec/1(Rr_LLCTemp_Nidec)  "<CAN3_Rr_LLCTemp_Nidec>"
  RrLLCTempNidec/1(VHAL_RrLLCTempNidec_C) -> VHAL_RrLLCTempNidec_C/1
  [DT_CAN3_SG_MCU_N_R2] -> bus_selector7/1
  bus_selector7/1 -> RrLLCflowReqNidec/1(Rr_LLCflowReq_Nidec)  "<CAN3_Rr_LLCflowReq_Nidec>"
  RrLLCflowReqNidec/1(VHAL_RrLLCflowReqNidec_Lpmin) -> VHAL_RrLLCflowReqNidec_Lpmin/1
  [DT_CAN3_SG_MCU_N_R2] -> bus_selector8/1
  bus_selector8/1 -> RrMCUTempWarnNidec/1(Rr_MCUTempWarn_Nidec)  "<CAN3_Rr_MCUTempWarn_Nidec>"
  RrMCUTempWarnNidec/1(VHAL_RrMCUTempWarnNidec_enum) -> VHAL_RrMCUTempWarnNidec_enum/1
  [DT_CAN3_SG_MCU_N_R2] -> bus_selector9/1
  bus_selector9/1 -> RrTMTempWarnNidec/1(Rr_TMTempWarn_Nidec)  "<CAN3_Rr_TMTempWarn_Nidec>"
  RrTMTempWarnNidec/1(VHAL_RrTMTempWarnNidec_enum) -> VHAL_RrTMTempWarnNidec_enum/1

== system halin/HAL_IN/CAN3/MCU_N_R3 ==
  DT_CAN3_SG_MCU_N_R3 : Inport
  RrMCU3HWVerNidec : Subsystem
  RrMCU3SWVerNidec : Subsystem
  bus_selector : BusSelector  OutputSignals=CAN3_Rr_MCU3_HW_Ver_Nidec
  bus_selector1 : BusSelector  OutputSignals=CAN3_Rr_MCU3_SW_Ver_Nidec
  VHAL_RrMCU3HWVerNidec_enum : Outport
  VHAL_RrMCU3SWVerNidec_enum : Outport  Port=2
  wires:
  DT_CAN3_SG_MCU_N_R3/1 -> [DT_CAN3_SG_MCU_N_R3]
  [DT_CAN3_SG_MCU_N_R3] -> bus_selector/1
  bus_selector/1 -> RrMCU3HWVerNidec/1(Rr_MCU3_HW_Ver_Nidec)  "<CAN3_Rr_MCU3_HW_Ver_Nidec>"
  RrMCU3HWVerNidec/1(VHAL_RrMCU3HWVerNidec_enum) -> VHAL_RrMCU3HWVerNidec_enum/1
  [DT_CAN3_SG_MCU_N_R3] -> bus_selector1/1
  bus_selector1/1 -> RrMCU3SWVerNidec/1(Rr_MCU3_SW_Ver_Nidec)  "<CAN3_Rr_MCU3_SW_Ver_Nidec>"
  RrMCU3SWVerNidec/1(VHAL_RrMCU3SWVerNidec_enum) -> VHAL_RrMCU3SWVerNidec_enum/1

== system halin/HAL_IN/CAN3/Shifter1 ==
  DT_CAN3_SG_Shifter1 : Inport
  0x9D : Constant  Value=0x9D
  0xF9 : Constant  Value=0xF9
  BitwiseAND{,1..3} (4 alike) : simulink/Logic and Bit Operations/Bitwise Operator  logicop=AND  UseBitMask=on  BitMask=0xFF  BitMaskRealWorld=Stored Integer
  BitwiseOR{,1..3} (4 alike) : simulink/Logic and Bit Operations/Bitwise Operator  logicop=OR  UseBitMask=off  BitMask=bin2dec('11011001')  BitMaskRealWorld=Stored Integer
  DDM_CS&RC_Comparison : FVT_lib/hal/DDM_CS&RC_Comparison  MsgCycleTime=100
  Data Type Conversion{,1..3} (4 alike) : DataTypeConversion  OutDataTypeStr=uint8
  KHAL_CAN3Shifter1E2E_flg : Constant  Value=KHAL_CAN3Shifter1E2E_flg
  LeftShift{,1..3} (4 alike) : ArithShift  BitShiftDirection=Left
  MessageRollingCounter : FVT_lib/hal/MessageRollingCounter  CounterMAX=14  task_time_ms=5  msg_time_ms=100
  Mux : Mux  Inputs=7
  ShifterCRC8 : Subsystem
  ShifterFailsta : Subsystem
  ShifterHandleCmd : Subsystem
  ShifterRC : Subsystem
  bus_selector : BusSelector  OutputSignals=CAN3_Shifter_CRC8,CAN3_Shifter_Fail_sta,CAN3_Shifter_Handle_Cmd,CAN3_Shifter_RC
  bus_selector1 : BusSelector  OutputSignals=CAN3_Shifter_CRC8
  bus_selector2 : BusSelector  OutputSignals=CAN3_Shifter_Fail_sta
  bus_selector3 : BusSelector  OutputSignals=CAN3_Shifter_Handle_Cmd
  bus_selector4 : BusSelector  OutputSignals=CAN3_Shifter_RC
  constant{,1..3} (4 alike) : Constant  Value=0x0  OutDataTypeStr=uint8
  VHAL_Shifter1CSErr_flg : Outport
  VHAL_Shifter1RCErr_flg : Outport  Port=2
  VHAL_ShifterCRC8_enum : Outport  Port=3
  VHAL_ShifterFailsta_enum : Outport  Port=4
  VHAL_ShifterHandleCmd_enum : Outport  Port=5
  VHAL_ShifterRC_enum : Outport  Port=6
  wires:
  DT_CAN3_SG_Shifter1/1 -> [DT_CAN3_SG_Shifter1]
  [DT_CAN3_SG_Shifter1] -> bus_selector/1
  bus_selector/1 -> [CAN3_Shifter_CRC8]  "<CAN3_Shifter_CRC8>"
  [CAN3_Shifter_CRC8] -> LeftShift/1
  LeftShift/1 -> BitwiseAND/1
  BitwiseAND/1 -> [Byte_0_CAN3_Shifter_CRC8]
  bus_selector/2 -> [CAN3_Shifter_Fail_sta]  "<CAN3_Shifter_Fail_sta>"
  [CAN3_Shifter_Fail_sta] -> LeftShift1/1
  LeftShift1/1 -> BitwiseAND1/1
  BitwiseAND1/1 -> [Byte_2_CAN3_Shifter_Fail_sta]
  bus_selector/3 -> [CAN3_Shifter_Handle_Cmd]  "<CAN3_Shifter_Handle_Cmd>"
  [CAN3_Shifter_Handle_Cmd] -> LeftShift2/1
  LeftShift2/1 -> BitwiseAND2/1
  BitwiseAND2/1 -> [Byte_7_CAN3_Shifter_Handle_Cmd]
  bus_selector/4 -> [CAN3_Shifter_RC]  "<CAN3_Shifter_RC>"
  [CAN3_Shifter_RC] -> LeftShift3/1
  LeftShift3/1 -> BitwiseAND3/1
  BitwiseAND3/1 -> [Byte_1_CAN3_Shifter_RC]
  Data Type Conversion/1 -> BitwiseOR/1
  [Byte_0_CAN3_Shifter_CRC8] -> Data Type Conversion/1
  BitwiseOR/1 -> [Byte_0]
  Data Type Conversion1/1 -> BitwiseOR1/1
  [Byte_1_CAN3_Shifter_RC] -> Data Type Conversion1/1
  BitwiseOR1/1 -> [Byte_1]
  Data Type Conversion2/1 -> BitwiseOR2/1
  [Byte_2_CAN3_Shifter_Fail_sta] -> Data Type Conversion2/1
  BitwiseOR2/1 -> [Byte_2]
  constant/1 -> [Byte_3]
  constant1/1 -> [Byte_4]
  constant2/1 -> [Byte_5]
  constant3/1 -> [Byte_6]
  Data Type Conversion3/1 -> BitwiseOR3/1
  [Byte_7_CAN3_Shifter_Handle_Cmd] -> Data Type Conversion3/1
  BitwiseOR3/1 -> [Byte_7]
  [Byte_1] -> Mux/1
  [Byte_2] -> Mux/2
  [Byte_3] -> Mux/3
  [Byte_4] -> Mux/4
  [Byte_5] -> Mux/5
  [Byte_6] -> Mux/6
  [Byte_7] -> Mux/7
  Mux/1 -> [VHAL_CAN3Shifter1noCS_raw]
  KHAL_CAN3Shifter1E2E_flg/1 -> DDM_CS&RC_Comparison/1
  0x9D/1 -> DDM_CS&RC_Comparison/2
  0xF9/1 -> DDM_CS&RC_Comparison/3
  [VHAL_CAN3Shifter1noCS_raw] -> DDM_CS&RC_Comparison/4
  [Byte_0] -> DDM_CS&RC_Comparison/5
  [RC_ECU] -> DDM_CS&RC_Comparison/6
  MessageRollingCounter/1 -> DDM_CS&RC_Comparison/7
  DDM_CS&RC_Comparison/1 -> VHAL_Shifter1CSErr_flg/1
  DDM_CS&RC_Comparison/2 -> VHAL_Shifter1RCErr_flg/1
  [DT_CAN3_SG_Shifter1] -> bus_selector1/1
  bus_selector1/1 -> ShifterCRC8/1(Shifter_CRC8)  "<CAN3_Shifter_CRC8>"
  ShifterCRC8/1(VHAL_ShifterCRC8_enum) -> VHAL_ShifterCRC8_enum/1
  [DT_CAN3_SG_Shifter1] -> bus_selector2/1
  bus_selector2/1 -> ShifterFailsta/1(Shifter_Fail_sta)  "<CAN3_Shifter_Fail_sta>"
  ShifterFailsta/1(VHAL_ShifterFailsta_enum) -> VHAL_ShifterFailsta_enum/1
  [DT_CAN3_SG_Shifter1] -> bus_selector3/1
  bus_selector3/1 -> ShifterHandleCmd/1(Shifter_Handle_Cmd)  "<CAN3_Shifter_Handle_Cmd>"
  ShifterHandleCmd/1(VHAL_ShifterHandleCmd_enum) -> VHAL_ShifterHandleCmd_enum/1
  [DT_CAN3_SG_Shifter1] -> bus_selector4/1
  bus_selector4/1 -> ShifterRC/1(Shifter_RC)  "<CAN3_Shifter_RC>"
  ShifterRC/1(VHAL_ShifterRC_enum) -> VHAL_ShifterRC_enum/1, [RC_ECU]

== system halin/HAL_IN/CAN3/Shifter2 ==
  DT_CAN3_SG_Shifter2 : Inport
  0x00 : Constant  Value=0x00
  0x1 : Constant  Value=0x00
  BitwiseAND{,1..5} (6 alike) : simulink/Logic and Bit Operations/Bitwise Operator  logicop=AND  UseBitMask=on  BitMask=0xFF  BitMaskRealWorld=Stored Integer
  BitwiseOR : simulink/Logic and Bit Operations/Bitwise Operator  logicop=OR  UseBitMask=off  NumInputPorts=3  BitMask=bin2dec('11011001')  BitMaskRealWorld=Stored Integer
  BitwiseOR1 : simulink/Logic and Bit Operations/Bitwise Operator  logicop=OR  UseBitMask=off  NumInputPorts=3  BitMask=bin2dec('11011001')  BitMaskRealWorld=Stored Integer
  CSW2DimSwSta : Subsystem
  CSW2FWasSwSta : Subsystem
  CSW2FWipSwSta : Subsystem
  CSW2PassSWSta : Subsystem
  CSW2RWipWasSwSta : Subsystem
  CSW2TurnSwSta : Subsystem
  DDM_CS&RC_Comparison : FVT_lib/hal/DDM_CS&RC_Comparison  MsgCycleTime=100
  Data Type Conversion{,1..5} (6 alike) : DataTypeConversion  OutDataTypeStr=uint8
  KHAL_CAN3Shifter2E2E_flg : Constant  Value=KHAL_CAN3Shifter2E2E_flg
  LeftShift : ArithShift  BitShiftNumber=7  BitShiftDirection=Left
  LeftShift1 : ArithShift  BitShiftDirection=Left
  LeftShift2 : ArithShift  BitShiftNumber=4  BitShiftDirection=Left
  LeftShift3 : ArithShift  BitShiftNumber=7  BitShiftDirection=Left
  LeftShift4 : ArithShift  BitShiftNumber=2  BitShiftDirection=Left
  LeftShift5 : ArithShift  BitShiftDirection=Left
  MessageRollingCounter : FVT_lib/hal/MessageRollingCounter  CounterMAX=14  task_time_ms=5  msg_time_ms=100
  Mux : Mux  Inputs=7
  bus_selector : BusSelector  OutputSignals=CAN3_CSW2_DimSw_Sta,CAN3_CSW2_FWasSw_Sta,CAN3_CSW2_FWipSw_Sta,CAN3_CSW2_PassSW_Sta,CAN3_CSW2_RWipWasSw_Sta,CAN3_CSW2_TurnSw_Sta
  bus_selector1 : BusSelector  OutputSignals=CAN3_CSW2_DimSw_Sta
  bus_selector2 : BusSelector  OutputSignals=CAN3_CSW2_FWasSw_Sta
  bus_selector3 : BusSelector  OutputSignals=CAN3_CSW2_FWipSw_Sta
  bus_selector4 : BusSelector  OutputSignals=CAN3_CSW2_PassSW_Sta
  bus_selector5 : BusSelector  OutputSignals=CAN3_CSW2_RWipWasSw_Sta
  bus_selector6 : BusSelector  OutputSignals=CAN3_CSW2_TurnSw_Sta
  constant{,1..5} (6 alike) : Constant  Value=0x0  OutDataTypeStr=uint8
  VHAL_Shifter2CSErr_flg : Outport
  VHAL_Shifter2RCErr_flg : Outport  Port=2
  VHAL_CSW2DimSwSta_flg : Outport  Port=3
  VHAL_CSW2FWasSwSta_enum : Outport  Port=4
  VHAL_CSW2FWipSwSta_enum : Outport  Port=5
  VHAL_CSW2PassSWSta_flg : Outport  Port=6
  VHAL_CSW2RWipWasSwSta_enum : Outport  Port=7
  VHAL_CSW2TurnSwSta_enum : Outport  Port=8
  wires:
  DT_CAN3_SG_Shifter2/1 -> [DT_CAN3_SG_Shifter2]
  [DT_CAN3_SG_Shifter2] -> bus_selector/1
  bus_selector/1 -> [CAN3_CSW2_DimSw_Sta]  "<CAN3_CSW2_DimSw_Sta>"
  [CAN3_CSW2_DimSw_Sta] -> LeftShift/1
  LeftShift/1 -> BitwiseAND/1
  BitwiseAND/1 -> [Byte_3_CAN3_CSW2_DimSw_Sta]
  bus_selector/2 -> [CAN3_CSW2_FWasSw_Sta]  "<CAN3_CSW2_FWasSw_Sta>"
  [CAN3_CSW2_FWasSw_Sta] -> LeftShift1/1
  LeftShift1/1 -> BitwiseAND1/1
  BitwiseAND1/1 -> [Byte_3_CAN3_CSW2_FWasSw_Sta]
  bus_selector/3 -> [CAN3_CSW2_FWipSw_Sta]  "<CAN3_CSW2_FWipSw_Sta>"
  [CAN3_CSW2_FWipSw_Sta] -> LeftShift2/1
  LeftShift2/1 -> BitwiseAND2/1
  BitwiseAND2/1 -> [Byte_2_CAN3_CSW2_FWipSw_Sta]
  bus_selector/4 -> [CAN3_CSW2_PassSW_Sta]  "<CAN3_CSW2_PassSW_Sta>"
  [CAN3_CSW2_PassSW_Sta] -> LeftShift3/1
  LeftShift3/1 -> BitwiseAND3/1
  BitwiseAND3/1 -> [Byte_2_CAN3_CSW2_PassSW_Sta]
  bus_selector/5 -> [CAN3_CSW2_RWipWasSw_Sta]  "<CAN3_CSW2_RWipWasSw_Sta>"
  [CAN3_CSW2_RWipWasSw_Sta] -> LeftShift4/1
  LeftShift4/1 -> BitwiseAND4/1
  BitwiseAND4/1 -> [Byte_3_CAN3_CSW2_RWipWasSw_Sta]
  bus_selector/6 -> [CAN3_CSW2_TurnSw_Sta]  "<CAN3_CSW2_TurnSw_Sta>"
  [CAN3_CSW2_TurnSw_Sta] -> LeftShift5/1
  LeftShift5/1 -> BitwiseAND5/1
  BitwiseAND5/1 -> [Byte_2_CAN3_CSW2_TurnSw_Sta]
  constant/1 -> [Byte_0]
  constant1/1 -> [Byte_1]
  Data Type Conversion/1 -> BitwiseOR/1
  [Byte_2_CAN3_CSW2_FWipSw_Sta] -> Data Type Conversion/1
  Data Type Conversion1/1 -> BitwiseOR/2
  [Byte_2_CAN3_CSW2_PassSW_Sta] -> Data Type Conversion1/1
  Data Type Conversion2/1 -> BitwiseOR/3
  [Byte_2_CAN3_CSW2_TurnSw_Sta] -> Data Type Conversion2/1
  BitwiseOR/1 -> [Byte_2]
  Data Type Conversion3/1 -> BitwiseOR1/1
  [Byte_3_CAN3_CSW2_DimSw_Sta] -> Data Type Conversion3/1
  Data Type Conversion4/1 -> BitwiseOR1/2
  [Byte_3_CAN3_CSW2_FWasSw_Sta] -> Data Type Conversion4/1
  Data Type Conversion5/1 -> BitwiseOR1/3
  [Byte_3_CAN3_CSW2_RWipWasSw_Sta] -> Data Type Conversion5/1
  BitwiseOR1/1 -> [Byte_3]
  constant2/1 -> [Byte_4]
  constant3/1 -> [Byte_5]
  constant4/1 -> [Byte_6]
  constant5/1 -> [Byte_7]
  [Byte_1] -> Mux/1
  [Byte_2] -> Mux/2
  [Byte_3] -> Mux/3
  [Byte_4] -> Mux/4
  [Byte_5] -> Mux/5
  [Byte_6] -> Mux/6
  [Byte_7] -> Mux/7
  Mux/1 -> [VHAL_CAN3Shifter2noCS_raw]
  KHAL_CAN3Shifter2E2E_flg/1 -> DDM_CS&RC_Comparison/1
  0x00/1 -> DDM_CS&RC_Comparison/2
  0x1/1 -> DDM_CS&RC_Comparison/3
  [VHAL_CAN3Shifter2noCS_raw] -> DDM_CS&RC_Comparison/4
  [Byte_0] -> DDM_CS&RC_Comparison/5
  [RC_ECU] -> DDM_CS&RC_Comparison/6
  MessageRollingCounter/1 -> DDM_CS&RC_Comparison/7
  DDM_CS&RC_Comparison/1 -> VHAL_Shifter2CSErr_flg/1
  DDM_CS&RC_Comparison/2 -> VHAL_Shifter2RCErr_flg/1
  [DT_CAN3_SG_Shifter2] -> bus_selector1/1
  bus_selector1/1 -> CSW2DimSwSta/1(CSW2_DimSw_Sta)  "<CAN3_CSW2_DimSw_Sta>"
  CSW2DimSwSta/1(VHAL_CSW2DimSwSta_flg) -> VHAL_CSW2DimSwSta_flg/1
  [DT_CAN3_SG_Shifter2] -> bus_selector2/1
  bus_selector2/1 -> CSW2FWasSwSta/1(CSW2_FWasSw_Sta)  "<CAN3_CSW2_FWasSw_Sta>"
  CSW2FWasSwSta/1(VHAL_CSW2FWasSwSta_enum) -> VHAL_CSW2FWasSwSta_enum/1
  [DT_CAN3_SG_Shifter2] -> bus_selector3/1
  bus_selector3/1 -> CSW2FWipSwSta/1(CSW2_FWipSw_Sta)  "<CAN3_CSW2_FWipSw_Sta>"
  CSW2FWipSwSta/1(VHAL_CSW2FWipSwSta_enum) -> VHAL_CSW2FWipSwSta_enum/1
  [DT_CAN3_SG_Shifter2] -> bus_selector4/1
  bus_selector4/1 -> CSW2PassSWSta/1(CSW2_PassSW_Sta)  "<CAN3_CSW2_PassSW_Sta>"
  CSW2PassSWSta/1(VHAL_CSW2PassSWSta_flg) -> VHAL_CSW2PassSWSta_flg/1
  [DT_CAN3_SG_Shifter2] -> bus_selector5/1
  bus_selector5/1 -> CSW2RWipWasSwSta/1(CSW2_RWipWasSw_Sta)  "<CAN3_CSW2_RWipWasSw_Sta>"
  CSW2RWipWasSwSta/1(VHAL_CSW2RWipWasSwSta_enum) -> VHAL_CSW2RWipWasSwSta_enum/1
  [DT_CAN3_SG_Shifter2] -> bus_selector6/1
  bus_selector6/1 -> CSW2TurnSwSta/1(CSW2_TurnSw_Sta)  "<CAN3_CSW2_TurnSw_Sta>"
  CSW2TurnSwSta/1(VHAL_CSW2TurnSwSta_enum) -> VHAL_CSW2TurnSwSta_enum/1

== system halin/HAL_IN/CAN3/VHAL_CANMsgInvalidBMS1_flg ==
  Cast To Boolean13 : DataTypeConversion  OutDataTypeStr=boolean
  Constant : Constant  Value=TRUE
  Latch13 : hcu_lib/Basic_Blocks/Latch
  Switch13 : Switch  Criteria=u2 ~= 0
  Unit Delay : UnitDelay  SampleTime=-1  HasFrameUpgradeWarning=on
  UnitConverter : DataTypeConversion  OutDataTypeStr=boolean
  Out : Outport
  wires:
  Constant/1 -> Switch13/3
  Unit Delay/1 -> Cast To Boolean13/1
  Cast To Boolean13/1 -> Switch13/1, Latch13/1
  Switch13/1 -> UnitConverter/1
  Latch13/1 -> Switch13/2
  UnitConverter/1 -> Unit Delay/1, Out/1  "VHAL_CANMsgInvalidBMS1_flg"

== system halin/HAL_IN/CAN3/VHAL_CANMsgInvalidBMS3_flg ==
  Cast To Boolean13 : DataTypeConversion  OutDataTypeStr=boolean
  Constant : Constant  Value=TRUE
  Latch13 : hcu_lib/Basic_Blocks/Latch
  Switch13 : Switch  Criteria=u2 ~= 0
  Unit Delay : UnitDelay  SampleTime=-1  HasFrameUpgradeWarning=on
  UnitConverter : DataTypeConversion  OutDataTypeStr=boolean
  Out : Outport
  wires:
  Constant/1 -> Switch13/3
  Unit Delay/1 -> Cast To Boolean13/1
  Cast To Boolean13/1 -> Switch13/1, Latch13/1
  Switch13/1 -> UnitConverter/1
  Latch13/1 -> Switch13/2
  UnitConverter/1 -> Unit Delay/1, Out/1  "VHAL_CANMsgInvalidBMS3_flg"

== system halin/HAL_IN/CAN3/VHAL_CANMsgInvalidBMS4_flg ==
  Cast To Boolean13 : DataTypeConversion  OutDataTypeStr=boolean
  Constant : Constant  Value=TRUE
  Latch13 : hcu_lib/Basic_Blocks/Latch
  Switch13 : Switch  Criteria=u2 ~= 0
  Unit Delay : UnitDelay  SampleTime=-1  HasFrameUpgradeWarning=on
  UnitConverter : DataTypeConversion  OutDataTypeStr=boolean
  Out : Outport
  wires:
  Constant/1 -> Switch13/3
  Unit Delay/1 -> Cast To Boolean13/1
  Cast To Boolean13/1 -> Switch13/1, Latch13/1
  Switch13/1 -> UnitConverter/1
  Latch13/1 -> Switch13/2
  UnitConverter/1 -> Unit Delay/1, Out/1  "VHAL_CANMsgInvalidBMS4_flg"

== system halin/HAL_IN/CAN3/VHAL_CANMsgInvalidBMS5_flg ==
  Cast To Boolean13 : DataTypeConversion  OutDataTypeStr=boolean
  Constant : Constant  Value=TRUE
  Latch13 : hcu_lib/Basic_Blocks/Latch
  Switch13 : Switch  Criteria=u2 ~= 0
  Unit Delay : UnitDelay  SampleTime=-1  HasFrameUpgradeWarning=on
  UnitConverter : DataTypeConversion  OutDataTypeStr=boolean
  Out : Outport
  wires:
  Constant/1 -> Switch13/3
  Unit Delay/1 -> Cast To Boolean13/1
  Cast To Boolean13/1 -> Switch13/1, Latch13/1
  Switch13/1 -> UnitConverter/1
  Latch13/1 -> Switch13/2
  UnitConverter/1 -> Unit Delay/1, Out/1  "VHAL_CANMsgInvalidBMS5_flg"

== system halin/HAL_IN/CAN3/VHAL_CANMsgInvalidBMS6_flg ==
  Cast To Boolean13 : DataTypeConversion  OutDataTypeStr=boolean
  Constant : Constant  Value=TRUE
  Latch13 : hcu_lib/Basic_Blocks/Latch
  Switch13 : Switch  Criteria=u2 ~= 0
  Unit Delay : UnitDelay  SampleTime=-1  HasFrameUpgradeWarning=on
  UnitConverter : DataTypeConversion  OutDataTypeStr=boolean
  Out : Outport
  wires:
  Constant/1 -> Switch13/3
  Unit Delay/1 -> Cast To Boolean13/1
  Cast To Boolean13/1 -> Switch13/1, Latch13/1
  Switch13/1 -> UnitConverter/1
  Latch13/1 -> Switch13/2
  UnitConverter/1 -> Unit Delay/1, Out/1  "VHAL_CANMsgInvalidBMS6_flg"

== system halin/HAL_IN/CAN3/VHAL_CANMsgInvalidBMS8_flg ==
  Cast To Boolean13 : DataTypeConversion  OutDataTypeStr=boolean
  Constant : Constant  Value=TRUE
  Latch13 : hcu_lib/Basic_Blocks/Latch
  Switch13 : Switch  Criteria=u2 ~= 0
  Unit Delay : UnitDelay  SampleTime=-1  HasFrameUpgradeWarning=on
  UnitConverter : DataTypeConversion  OutDataTypeStr=boolean
  Out : Outport
  wires:
  Constant/1 -> Switch13/3
  Unit Delay/1 -> Cast To Boolean13/1
  Cast To Boolean13/1 -> Switch13/1, Latch13/1
  Switch13/1 -> UnitConverter/1
  Latch13/1 -> Switch13/2
  UnitConverter/1 -> Unit Delay/1, Out/1  "VHAL_CANMsgInvalidBMS8_flg"

== system halin/HAL_IN/CAN3/VHAL_CANMsgInvalidCCU1_flg ==
  Cast To Boolean13 : DataTypeConversion  OutDataTypeStr=boolean
  Constant : Constant  Value=TRUE
  Latch13 : hcu_lib/Basic_Blocks/Latch
  Switch13 : Switch  Criteria=u2 ~= 0
  Unit Delay : UnitDelay  SampleTime=-1  HasFrameUpgradeWarning=on
  UnitConverter : DataTypeConversion  OutDataTypeStr=boolean
  Out : Outport
  wires:
  Constant/1 -> Switch13/3
  Unit Delay/1 -> Cast To Boolean13/1
  Cast To Boolean13/1 -> Switch13/1, Latch13/1
  Switch13/1 -> UnitConverter/1
  Latch13/1 -> Switch13/2
  UnitConverter/1 -> Unit Delay/1, Out/1  "VHAL_CANMsgInvalidCCU1_flg"

== system halin/HAL_IN/CAN3/VHAL_CANMsgInvalidCCU2_flg ==
  Cast To Boolean13 : DataTypeConversion  OutDataTypeStr=boolean
  Constant : Constant  Value=TRUE
  Latch13 : hcu_lib/Basic_Blocks/Latch
  Switch13 : Switch  Criteria=u2 ~= 0
  Unit Delay : UnitDelay  SampleTime=-1  HasFrameUpgradeWarning=on
  UnitConverter : DataTypeConversion  OutDataTypeStr=boolean
  Out : Outport
  wires:
  Constant/1 -> Switch13/3
  Unit Delay/1 -> Cast To Boolean13/1
  Cast To Boolean13/1 -> Switch13/1, Latch13/1
  Switch13/1 -> UnitConverter/1
  Latch13/1 -> Switch13/2
  UnitConverter/1 -> Unit Delay/1, Out/1  "VHAL_CANMsgInvalidCCU2_flg"

== system halin/HAL_IN/CAN3/VHAL_CANMsgInvalidEBM1_flg ==
  Cast To Boolean13 : DataTypeConversion  OutDataTypeStr=boolean
  Constant : Constant  Value=TRUE
  Latch13 : hcu_lib/Basic_Blocks/Latch
  Switch13 : Switch  Criteria=u2 ~= 0
  Unit Delay : UnitDelay  SampleTime=-1  HasFrameUpgradeWarning=on
  UnitConverter : DataTypeConversion  OutDataTypeStr=boolean
  Out : Outport
  wires:
  Constant/1 -> Switch13/3
  Unit Delay/1 -> Cast To Boolean13/1
  Cast To Boolean13/1 -> Switch13/1, Latch13/1
  Switch13/1 -> UnitConverter/1
  Latch13/1 -> Switch13/2
  UnitConverter/1 -> Unit Delay/1, Out/1  "VHAL_CANMsgInvalidEBM1_flg"

== system halin/HAL_IN/CAN3/VHAL_CANMsgInvalidMCUBF1_flg ==
  Cast To Boolean13 : DataTypeConversion  OutDataTypeStr=boolean
  Constant : Constant  Value=TRUE
  Latch13 : hcu_lib/Basic_Blocks/Latch
  Switch13 : Switch  Criteria=u2 ~= 0
  Unit Delay : UnitDelay  SampleTime=-1  HasFrameUpgradeWarning=on
  UnitConverter : DataTypeConversion  OutDataTypeStr=boolean
  Out : Outport
  wires:
  Constant/1 -> Switch13/3
  Unit Delay/1 -> Cast To Boolean13/1
  Cast To Boolean13/1 -> Switch13/1, Latch13/1
  Switch13/1 -> UnitConverter/1
  Latch13/1 -> Switch13/2
  UnitConverter/1 -> Unit Delay/1, Out/1  "VHAL_CANMsgInvalidMCUBF1_flg"

== system halin/HAL_IN/CAN3/VHAL_CANMsgInvalidMCUBF2_flg ==
  Cast To Boolean13 : DataTypeConversion  OutDataTypeStr=boolean
  Constant : Constant  Value=TRUE
  Latch13 : hcu_lib/Basic_Blocks/Latch
  Switch13 : Switch  Criteria=u2 ~= 0
  Unit Delay : UnitDelay  SampleTime=-1  HasFrameUpgradeWarning=on
  UnitConverter : DataTypeConversion  OutDataTypeStr=boolean
  Out : Outport
  wires:
  Constant/1 -> Switch13/3
  Unit Delay/1 -> Cast To Boolean13/1
  Cast To Boolean13/1 -> Switch13/1, Latch13/1
  Switch13/1 -> UnitConverter/1
  Latch13/1 -> Switch13/2
  UnitConverter/1 -> Unit Delay/1, Out/1  "VHAL_CANMsgInvalidMCUBF2_flg"

== system halin/HAL_IN/CAN3/VHAL_CANMsgInvalidMCUBR1_flg ==
  Cast To Boolean13 : DataTypeConversion  OutDataTypeStr=boolean
  Constant : Constant  Value=TRUE
  Latch13 : hcu_lib/Basic_Blocks/Latch
  Switch13 : Switch  Criteria=u2 ~= 0
  Unit Delay : UnitDelay  SampleTime=-1  HasFrameUpgradeWarning=on
  UnitConverter : DataTypeConversion  OutDataTypeStr=boolean
  Out : Outport
  wires:
  Constant/1 -> Switch13/3
  Unit Delay/1 -> Cast To Boolean13/1
  Cast To Boolean13/1 -> Switch13/1, Latch13/1
  Switch13/1 -> UnitConverter/1
  Latch13/1 -> Switch13/2
  UnitConverter/1 -> Unit Delay/1, Out/1  "VHAL_CANMsgInvalidMCUBR1_flg"

== system halin/HAL_IN/CAN3/VHAL_CANMsgInvalidMCUBR2_flg ==
  Cast To Boolean13 : DataTypeConversion  OutDataTypeStr=boolean
  Constant : Constant  Value=TRUE
  Latch13 : hcu_lib/Basic_Blocks/Latch
  Switch13 : Switch  Criteria=u2 ~= 0
  Unit Delay : UnitDelay  SampleTime=-1  HasFrameUpgradeWarning=on
  UnitConverter : DataTypeConversion  OutDataTypeStr=boolean
  Out : Outport
  wires:
  Constant/1 -> Switch13/3
  Unit Delay/1 -> Cast To Boolean13/1
  Cast To Boolean13/1 -> Switch13/1, Latch13/1
  Switch13/1 -> UnitConverter/1
  Latch13/1 -> Switch13/2
  UnitConverter/1 -> Unit Delay/1, Out/1  "VHAL_CANMsgInvalidMCUBR2_flg"
